simulink model "model_par_gb_2018a"  (Simulink 10.1)
settings: Solver=VariableStepAuto  StartTime=0.0  StopTime=200  FixedStep=1  RelTol=1e-6
undefined symbols (not defined in the file or in its folder): alfa, beta1, beta2, beta3, beta4, d1, d2, d3, delta1, delta2, delta3, delta4, starting_pop, test_ratio, v1, v2, v3
settings Model: Creator=Piotr  LastModifiedBy=Piotr
settings DataIOCC: ReturnWorkspaceOutputs=on
settings OptimizationCC: LifeSpan=auto
settings DebuggingCC: UnderspecifiedInitializationDetection=Simplified  MergeDetectMultiDrivingBlocksExec=error  SFUnexpectedBacktrackingDiag=error  SFNoUnconditionalDefaultTransitionDiag=error  SFExecutionAtInitializationDiag=warning
settings HardwareCC: ProdBitPerPointer=64  ProdBitPerSizeT=64  ProdBitPerPtrDiffT=64  ProdLargestAtomicFloat=Float  ProdIntDivRoundTo=Zero  ProdEndianess=LittleEndian  ProdWordSize=64  ProdHWDeviceType=Intel->x86-64 (Windows64)
settings ModelReferenceCC: PropagateSignalLabelsOutOfModel=on
settings SFSimCC: SimUseLocalCustomCode=on
settings RTWCC: RTWUseLocalCustomCode=on
settings CodeAppCC: StateflowObjectComments=off
settings GRTTargetCC: TargetLangStandard=C99 (ISO)  CombineOutputUpdateFcns=on  GRTInterface=off
settings ConfigComp: CovMetricSettings=dwe  CovHtmlReporting=off  CovSaveCumulativeToWorkspaceVar=off  CovSaveSingleToWorkspaceVar=off  CovExternalEMLEnable=on

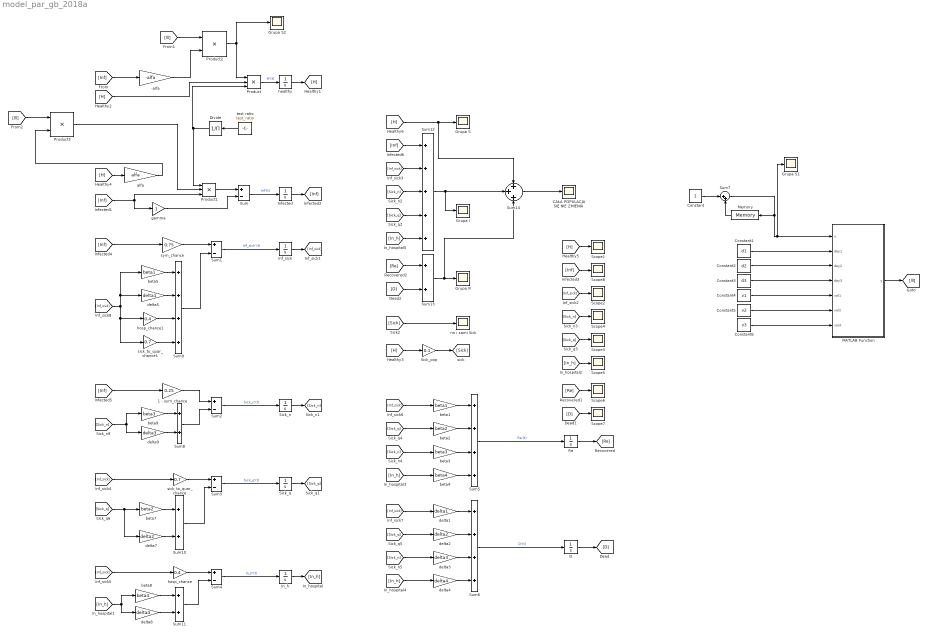
== system model_par_gb_2018a ==
  -alfa : Gain  Gain=-alfa
  1 - sym_chance : Gain  Gain=0.25
  CAŁA POPULACJA SIĘ NIE ZMIENIA : Scope
  Constant : Constant
  Constant1 : Constant  Value=d1
  Constant2 : Constant  Value=d2
  Constant3 : Constant  Value=d3
  Constant4 : Constant  Value=v1
  Constant5 : Constant  Value=v2
  Constant6 : Constant  Value=v3
  D : Integrator
  Divide : Product  Inputs=/
  Grupa I : Scope
  Grupa R : Scope
  Grupa S : Scope
  Grupa S1 : Scope
  Grupa S2 : Scope
  In_h : Integrator
  Inf_sick : Integrator
  Infected : Integrator  InitialCondition=10
  MATLAB Function : MATLAB Function  TreatAsAtomicUnit=on
  Memory : Memory
  Product : Product  Inputs=3
  Product1 : Product  Inputs=3
  Product2 : Product
  Product3 : Product
  Re : Integrator
  Scope{1..8} (8 alike) : Scope
  Sick_n : Integrator
  Sick_pop : Gain  Gain=0.1
  Sick_q : Integrator
  Sum{,1..4} (5 alike) : Sum  Inputs=+-
  Sum{8,10..11,13} (4 alike) : Sum
  Sum12 : Sum  Inputs=+++++
  Sum14 : Sum  Inputs=+++
  Sum5 : Sum  Inputs=++++
  Sum6 : Sum  Inputs=++++
  Sum7 : Sum  Inputs=|++
  Sum9 : Sum  Inputs=++++
  alfa : Gain  Gain=alfa
  beta1 : Gain  Gain=beta1
  beta2 : Gain  Gain=beta2
  beta3 : Gain  Gain=beta3
  beta4 : Gain  Gain=beta4
  beta5 : Gain  Gain=beta1
  beta7 : Gain  Gain=beta2
  beta8 : Gain  Gain=beta4
  beta9 : Gain  Gain=beta3
  delta1 : Gain  Gain=delta1
  delta2 : Gain  Gain=delta2
  delta3 : Gain  Gain=delta3
  delta4 : Gain  Gain=delta4
  delta5 : Gain  Gain=delta1
  delta7 : Gain  Gain=delta2
  delta8 : Gain  Gain=delta4
  delta9 : Gain  Gain=delta3
  gamma : Gain
  healthy : Integrator  InitialCondition=starting_pop
  hosp_chance : Gain  Gain=0.4
  hosp_chance1 : Gain  Gain=0.4
  no i sami Sick : Scope
  sick_to_quar_chance : Gain  Gain=0.7
  sick_to_quar_chance1 : Gain  Gain=0.7
  sym_chance : Gain  Gain=0.75
  test ratio : Constant  Value=test_ratio
  wires:
  healthy/1 -> [H]
  -alfa/1 -> Product2/2
  [Inf] -> -alfa/1
  Product/1 -> healthy/1  "H'(t)"
  [H] -> Product/2
  [H] -> Sick_pop/1
  Sick_pop/1 -> [Sick]
  Sum/1 -> Infected/1  "Inf'(t)"
  [Inf] -> Product1/3, gamma/1
  gamma/1 -> Sum/2
  [H] -> alfa/1
  Product1/1 -> Sum/1
  Infected/1 -> [Inf]
  [Inf] -> sym_chance/1
  sym_chance/1 -> Sum1/1
  Sum1/1 -> Inf_sick/1  "Inf_sick'(t)"
  Inf_sick/1 -> [Inf_sick]
  Sum2/1 -> Sick_n/1  "Sick_n'(t)"
  Sick_n/1 -> [Sick_n]
  1 - sym_chance/1 -> Sum2/1
  [Inf] -> 1 - sym_chance/1
  Sum3/1 -> Sick_q/1  "Sick_q'(t)"
  Sick_q/1 -> [Sick_q]
  sick_to_quar_chance/1 -> Sum3/1
  Sum4/1 -> In_h/1  "In_h'(t)"
  In_h/1 -> [In_h]
  hosp_chance/1 -> Sum4/1
  beta2/1 -> Sum5/2
  beta1/1 -> Sum5/1
  beta3/1 -> Sum5/3
  Sum5/1 -> Re/1  "Re'(t)"
  Re/1 -> [Re]
  beta4/1 -> Sum5/4
  delta2/1 -> Sum6/2
  delta4/1 -> Sum6/4
  Sum6/1 -> D/1  "D'(t)"
  delta3/1 -> Sum6/3
  delta1/1 -> Sum6/1
  D/1 -> [D]
  [Inf_sick] -> beta5/1, delta5/1, hosp_chance1/1, sick_to_quar_chance1/1
  [Inf_sick] -> beta1/1
  [Sick_q] -> beta2/1
  [Sick_n] -> beta3/1
  [Inf_sick] -> delta1/1
  [Sick_q] -> delta2/1
  [Sick_n] -> delta3/1
  [In_h] -> delta4/1
  [Inf_sick] -> hosp_chance/1
  [Sick_q] -> beta7/1, delta7/1
  [Inf_sick] -> sick_to_quar_chance/1
  [In_h] -> beta4/1
  [In_h] -> beta8/1, delta8/1
  [Sick_n] -> delta9/1, beta9/1
  beta9/1 -> Sum8/1
  delta9/1 -> Sum8/2
  Sum8/1 -> Sum2/2
  beta5/1 -> Sum9/1
  delta5/1 -> Sum9/2
  hosp_chance1/1 -> Sum9/3
  sick_to_quar_chance1/1 -> Sum9/4
  Sum9/1 -> Sum1/2
  beta7/1 -> Sum10/1
  delta7/1 -> Sum10/2
  Sum10/1 -> Sum3/2
  beta8/1 -> Sum11/1
  delta8/1 -> Sum11/2
  Sum11/1 -> Sum4/2
  [H] -> Sum14/1, Grupa S/1
  [Inf] -> Sum12/1
  [Inf_sick] -> Sum12/2
  [Sick_n] -> Sum12/3
  [Sick_q] -> Sum12/4
  [In_h] -> Sum12/5
  Sum12/1 -> Sum14/2, Grupa I/1
  [Re] -> Sum13/1
  [D] -> Sum13/2
  Sum13/1 -> Sum14/3, Grupa R/1
  Sum14/1 -> CAŁA POPULACJA SIĘ NIE ZMIENIA/1
  [Sick] -> no i sami Sick/1
  [Inf_sick] -> Scope2/1
  [Sick_n] -> Scope4/1
  [Sick_q] -> Scope3/1
  [In_h] -> Scope5/1
  [Re] -> Scope6/1
  [D] -> Scope7/1
  [Inf] -> Scope8/1
  [H] -> Scope1/1
  test ratio/1 -> Divide/1
  Divide/1 -> Product/3, Product1/1
  Memory/1 -> Sum7/2
  Constant/1 -> Sum7/1
  Product2/1 -> Product/1, Grupa S2/1
  Sum7/1 -> MATLAB Function/1(u), Grupa S1/1, Memory/1
  [lll] -> Product2/1
  Product3/1 -> Product1/2
  alfa/1 -> Product3/2
  [lll] -> Product3/1
  MATLAB Function/1(y) -> [lll]
  Constant1/1 -> MATLAB Function/2(day1)
  Constant2/1 -> MATLAB Function/3(day2)
  Constant3/1 -> MATLAB Function/4(day3)
  Constant4/1 -> MATLAB Function/5(val1)
  Constant5/1 -> MATLAB Function/6(val2)
  Constant6/1 -> MATLAB Function/7(val3)

== matlab function MATLAB Function ==
  data: u input double; y output double; day1 input double; day2 input double; day3 input double; val1 input double; val2 input double; val3 input double
function y = ref_fun(u,day1,day2,day3,val1,val2,val3)

if u >= day1 && (u < day2|| day2 == 0) && day1 ~= 0 
    y = val1;
elseif u >= day2 && (u < day3|| day3 == 0) && day2 ~= 0 
    y = val2;
elseif u >= day3 && day3 ~= 0
    y = val3;
else 
    y = 1;
end
end
